simulink model "vRTHS_MDOF_SimRT"  (R2016a)
settings: Solver=ode4  StartTime=0.0  StopTime=tend  FixedStep=dt_rths  RelTol=1e-3
values from neighbouring files (symbols this model uses):
  a = 53354    [A3_Frequency_Response.m]    (also in F2_controller.m)
  a1_beta0 = 2.1283e+13    (= 21283000000000)    [F1_input_file.m]
  a2 = 4.23e6    (= 4230000)    [A3_Frequency_Response.m]    (also in F1_input_file.m = 4229700)
  a3 = [3.3-uncer*1.3,3.3+uncer*1.3]    [A3_Frequency_Response.m]    (also in F1_input_file.m = 3.3        + 1.3   * nom *randn(1,1))
  A_ns = [     zeros(n) eye(n) ... (first row only)    [F1_input_file.m]
  Ax = [0 1;-c -b]    [F2_controller.m]
  B_ns = [     zeros(n,1)      zeros(n) ... (first row only)    [F1_input_file.m]
  beta1 = 425        + 3.3   * nom *randn(1,1)    [F1_input_file.m]
  beta2 = 9.9976e+04 + 3.3e3 * nom *randn(1,1)    [F1_input_file.m]
  Bx = [0;1]    [F2_controller.m]
  C_ns = [     eye(n)              zeros(n) ... (first row only)    [F1_input_file.m]
  CE = zeros(n)    [F1_input_file.m]
  compd = [dt_rths 1]    [F2_controller.m]
  compn = [2*dt_rths 1]    [F2_controller.m]
  Cx = [1,0]    [F2_controller.m]
  d = 0.00010595    [A3_Frequency_Response.m]    (also in F2_controller.m)
  D_ns = [     zeros(n,1)      zeros(n) ... (first row only)    [F1_input_file.m]
  dt_rths = 1/fs    (= 0.000244140625)    [A1_main_SMC.m]    (also in A2_main_PI.m; A4_Plots.m)
  Dx = 0    [F2_controller.m]
  E_sw = 1    [A4_Plots.m]
  eq_intensity = .4    (= 0.4)    [A1_main_SMC.m]    (also in A2_main_PI.m; A4_Plots.m)
  Gsnsr_DT = 1    [F1_input_file.m]
  Gsnsr_FT = 1    [F1_input_file.m]
  KE = zeros(n)    [F1_input_file.m]
  ME = zeros(n)    [F1_input_file.m]
  Para = [b c b*bc c*cc lambda eta sw]    [F2_controller.m]
  Rx = rms_noise_DT/dt_rths    [F2_controller.m]
  Seed_snr = rng(seed)    [F1_input_file.m]
  tend = 90    [F1_input_file.m]
  xinitial = zeros(2,1)    [F2_controller.m]
undefined symbols (not defined in the file or in its folder): Continuous, Time
libraries: simulink x3, ctrlSharedLib x1, sldrtlib x1
settings Model: Creator=IISL_0175  LastModifiedBy=user
settings DataIOCC: SaveFormat=StructureWithTime
settings DebuggingCC: InheritedTsInSrcMsg=none
settings HardwareCC: ProdWordSize=32  ProdHWDeviceType=Specified

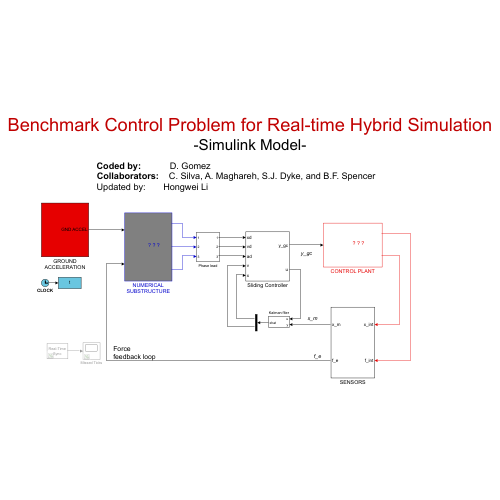
[thumbnail: Simulink's stored preview of the top-level diagram]
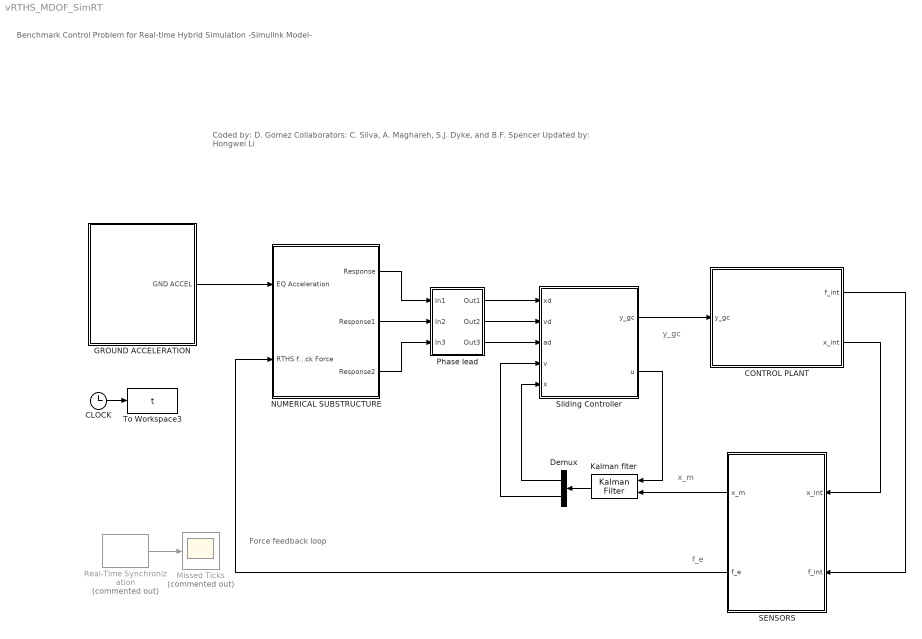
== system vRTHS_MDOF_SimRT ==
  note: Force
      | feedback loop
  note: Benchmark Control Problem for Real-time Hybrid Simulation
      | -Simulink Model-
  note: Coded by: D. Gomez
      | Collaborators: C. Silva, A. Maghareh, S.J. Dyke, and B.F. Spencer
      | Updated by: Hongwei Li
  note: y_gc
  note: f_e
  note: x_m
  CLOCK : Clock
  CONTROL PLANT : Subsystem
      mask Display: image(imread('PlantSW2.PNG'));
  Demux : Demux  Outputs=2
  GROUND ACCELERATION : Subsystem
  Kalman flter : ctrlSharedLib/Kalman Filter  TimeDomain=Continuous-Time  UseCurrentEstimator=on  ModelSource=Individual A, B, C, D matrices  ModelSourceVariable=ss(0.95,1,1,0,1)  A=Ax  B=Bx  C=Cx  D=Dx  NumberOfStates=2  NumberOfInputs=2  NumberOfOutputs=1  InitialEstimateSource=Dialog  X0=xinitial  P0=10  UseK=off  UseGH=off  NumberOfProcessNoiseInputs=1  G=1  TimeInvariantG=on  H=0  TimeInvariantH=on  Q=0  TimeInvariantQ=on  R=Rx  TimeInvariantR=on  N=0  TimeInvariantN=on  AddInputPort=on  AddEnablePort=off  OutputEstimatedY=off  OutputP=off  Ts=-1
  Missed Ticks : Scope  Commented=on
  NUMERICAL SUBSTRUCTURE : Subsystem
      mask Display: image(imread('Num_sub.png'));
  Phase lead : Subsystem
  Real-Time Synchronization : sldrtlib/Real-Time Synchronization  Commented=on  SampleTime=dt_rths  MaxMissedTicks=10000  ShowMissedTicks=on  YieldWhenWaiting=off
  SENSORS : Subsystem
  Sliding Controller : Subsystem
  To Workspace3 : ToWorkspace  VariableName=t  SampleTime=-1
  wires:
  CLOCK/1 -> To Workspace3/1
  CONTROL PLANT/2(x_int) -> SENSORS/1(x_int)
  Sliding Controller/1(y_gc) -> CONTROL PLANT/1(y_gc)
  Real-Time Synchronization/1 -> Missed Ticks/1
  GROUND ACCELERATION/1(GND ACCEL) -> NUMERICAL SUBSTRUCTURE/1(EQ Acceleration)
  CONTROL PLANT/1(f_int) -> SENSORS/2(f_int)
  SENSORS/2("f_e ") -> NUMERICAL SUBSTRUCTURE/2(RTHS feedback Force)
  NUMERICAL SUBSTRUCTURE/1(Response) -> Phase lead/1(In1)
  Phase lead/1(Out1) -> Sliding Controller/1(xd)
  Phase lead/2(Out2) -> Sliding Controller/2(vd)
  Phase lead/3(Out3) -> Sliding Controller/3(ad)
  NUMERICAL SUBSTRUCTURE/2(Response1) -> Phase lead/2(In2)
  NUMERICAL SUBSTRUCTURE/3(Response2) -> Phase lead/3(In3)
  Demux/1 -> Sliding Controller/5(x)
  Kalman flter/1 -> Demux/1
  SENSORS/1(x_m) -> Kalman flter/2
  Sliding Controller/2(u) -> Kalman flter/1
  Demux/2 -> Sliding Controller/4(v)

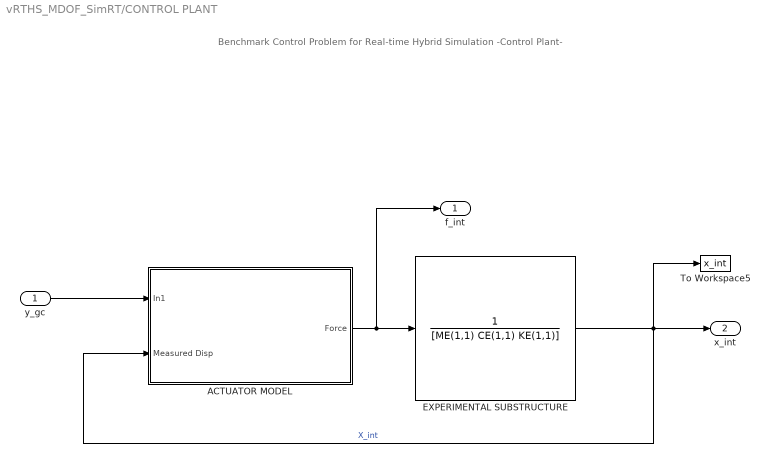
== system vRTHS_MDOF_SimRT/CONTROL PLANT ==
  note: Benchmark Control Problem for Real-time Hybrid Simulation
      | -Control Plant-
  y_gc : Inport
  ACTUATOR MODEL : Subsystem
      mask Display: image(imread('ActuatorSW2.PNG'));
  EXPERIMENTAL SUBSTRUCTURE : TransferFcn  Numerator=1  Denominator=[ME(1,1) CE(1,1) KE(1,1)]
      mask Display: image(imread('ESSW2.PNG'));
  To Workspace5 : ToWorkspace  VariableName=x_int  SampleTime=-1
  f_int : Outport
  x_int : Outport  Port=2
  wires:
  EXPERIMENTAL SUBSTRUCTURE/1 -> ACTUATOR MODEL/2(Measured Disp), To Workspace5/1, x_int/1  "X_int"
  ACTUATOR MODEL/1(Force) -> f_int/1, EXPERIMENTAL SUBSTRUCTURE/1
  y_gc/1 -> ACTUATOR MODEL/1(In1)

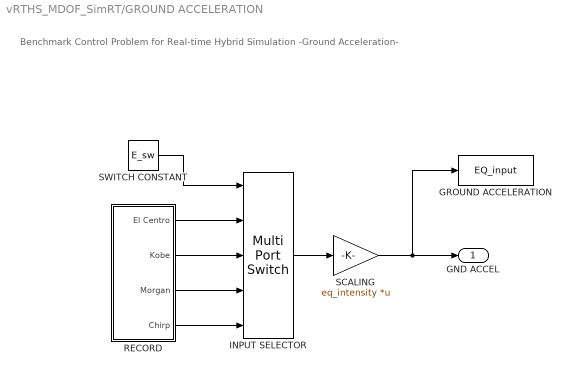
== system vRTHS_MDOF_SimRT/GROUND ACCELERATION ==
  note: Benchmark Control Problem for Real-time Hybrid Simulation
      | -Ground Acceleration-
  GROUND ACCELERATION : ToWorkspace  VariableName=EQ_input  SampleTime=-1
  INPUT SELECTOR : MultiPortSwitch  Inputs=4
  "RECORD " : Subsystem
  SCALING : Gain  Gain=eq_intensity  Multiplication=Matrix(K*u)
  SWITCH CONSTANT : Constant  Value=E_sw
  GND ACCEL : Outport
  wires:
  INPUT SELECTOR/1 -> SCALING/1
  SWITCH CONSTANT/1 -> INPUT SELECTOR/1
  "RECORD "/1(El Centro) -> INPUT SELECTOR/2
  "RECORD "/2(Kobe) -> INPUT SELECTOR/3
  "RECORD "/3(Morgan) -> INPUT SELECTOR/4
  SCALING/1 -> GROUND ACCELERATION/1, GND ACCEL/1
  "RECORD "/4(Chirp) -> INPUT SELECTOR/5

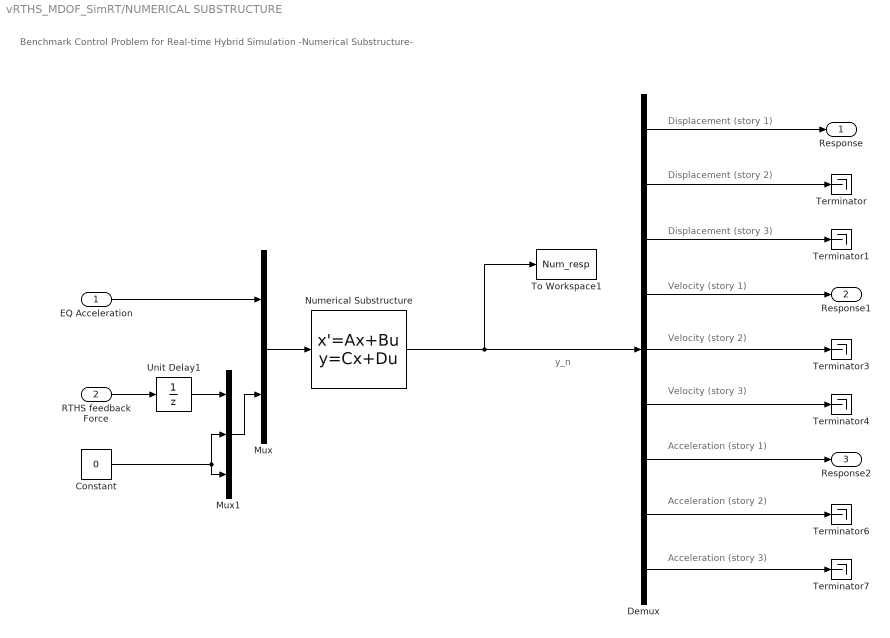
== system vRTHS_MDOF_SimRT/NUMERICAL SUBSTRUCTURE ==
  note: y_n
  note: Benchmark Control Problem for Real-time Hybrid Simulation
      | -Numerical Substructure-
  note: Velocity (story 3)
  note: Displacement (story 3)
  note: Displacement (story 1)
  note: Acceleration (story 1)
  note: Velocity (story 1)
  note: Velocity (story 2)
  note: Acceleration (story 3)
  note: Displacement (story 2)
  note: Acceleration (story 2)
  EQ Acceleration : Inport
  RTHS feedback Force : Inport  Port=2
  Constant : Constant  Value=0
  Demux : Demux  Outputs=9
  Mux : Mux  Inputs=2
  Mux1 : Mux  Inputs=3
  Numerical Substructure : StateSpace  A=A_ns  B=B_ns  C=C_ns  D=D_ns  X0=0
  Terminator{,1,3..4,6..7} (6 alike) : Terminator
  To Workspace1 : ToWorkspace  VariableName=Num_resp  SaveFormat=Timeseries  SampleTime=-1
  Unit Delay1 : UnitDelay  SampleTime=-1  HasFrameUpgradeWarning=on
  Response : Outport
  Response1 : Outport  Port=2
  Response2 : Outport  Port=3
  wires:
  Mux/1 -> Numerical Substructure/1
  EQ Acceleration/1 -> Mux/1
  RTHS feedback Force/1 -> Unit Delay1/1
  Numerical Substructure/1 -> To Workspace1/1, Demux/1
  Demux/2 -> Terminator/1
  Demux/7 -> Response2/1
  Demux/8 -> Terminator6/1
  Demux/9 -> Terminator7/1
  Demux/4 -> Response1/1
  Demux/6 -> Terminator4/1
  Demux/5 -> Terminator3/1
  Demux/1 -> Response/1
  Demux/3 -> Terminator1/1
  Constant/1 -> Mux1/2, Mux1/3
  Mux1/1 -> Mux/2
  Unit Delay1/1 -> Mux1/1

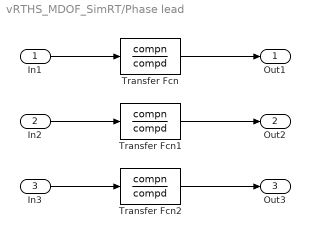
== system vRTHS_MDOF_SimRT/Phase lead ==
  In1 : Inport
  In2 : Inport  Port=2
  In3 : Inport  Port=3
  Transfer Fcn : TransferFcn  Numerator=compn  Denominator=compd
  Transfer Fcn1 : TransferFcn  Numerator=compn  Denominator=compd
  Transfer Fcn2 : TransferFcn  Numerator=compn  Denominator=compd
  Out1 : Outport
  Out2 : Outport  Port=2
  Out3 : Outport  Port=3
  wires:
  In1/1 -> Transfer Fcn/1
  Transfer Fcn/1 -> Out1/1
  In2/1 -> Transfer Fcn1/1
  Transfer Fcn1/1 -> Out2/1
  In3/1 -> Transfer Fcn2/1
  Transfer Fcn2/1 -> Out3/1

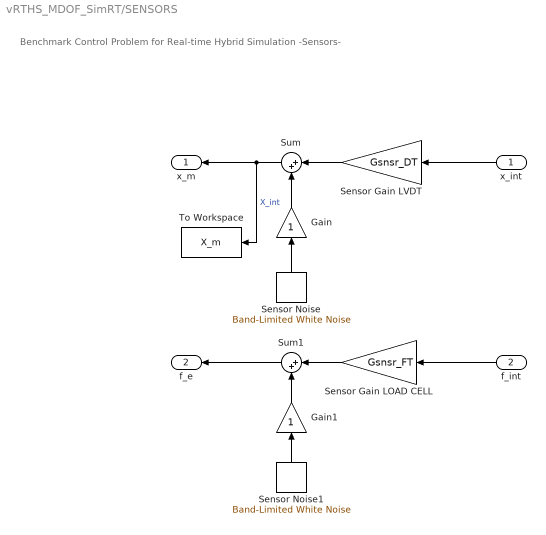
== system vRTHS_MDOF_SimRT/SENSORS ==
  note: Benchmark Control Problem for Real-time Hybrid Simulation
      | -Sensors-
  x_int : Inport
  f_int : Inport  Port=2
  Gain : Gain
  Gain1 : Gain
  Sensor Noise : simulink/Sources/Band-Limited White Noise  Cov=rms_noise_DT  Ts=dt_rths  seed=double(Seed_snr.Seed)
  Sensor Noise1 : simulink/Sources/Band-Limited White Noise  Cov=rms_noise_FT  Ts=dt_rths  seed=double(Seed_snr.Seed)
  Sensor Gain LVDT : Gain  Gain=Gsnsr_DT  SaturateOnIntegerOverflow=on  OutDataTypeStr=Inherit: Same as input  ParamDataTypeStr=Inherit: Same as input
  Sensor Gain LOAD CELL : Gain  Gain=Gsnsr_FT  SaturateOnIntegerOverflow=on  OutDataTypeStr=Inherit: Same as input  ParamDataTypeStr=Inherit: Same as input
  Sum : Sum  Inputs=|++  InputSameDT=on  SaturateOnIntegerOverflow=on  OutDataTypeStr=Inherit: Same as first input
  Sum1 : Sum  Inputs=|++  InputSameDT=on  SaturateOnIntegerOverflow=on  OutDataTypeStr=Inherit: Same as first input
  To Workspace : ToWorkspace  VariableName=X_m  SaveFormat=Timeseries  SampleTime=-1
  x_m : Outport
  "f_e " : Outport  Port=2
  wires:
  Sensor Gain LVDT/1 -> Sum/1
  Sensor Noise/1 -> Gain/1
  x_int/1 -> Sensor Gain LVDT/1
  Sensor Gain LOAD CELL/1 -> Sum1/1
  Sum1/1 -> "f_e "/1
  Sensor Noise1/1 -> Gain1/1
  f_int/1 -> Sensor Gain LOAD CELL/1
  Sum/1 -> x_m/1, To Workspace/1  "X_int"
  Gain/1 -> Sum/2
  Gain1/1 -> Sum1/2

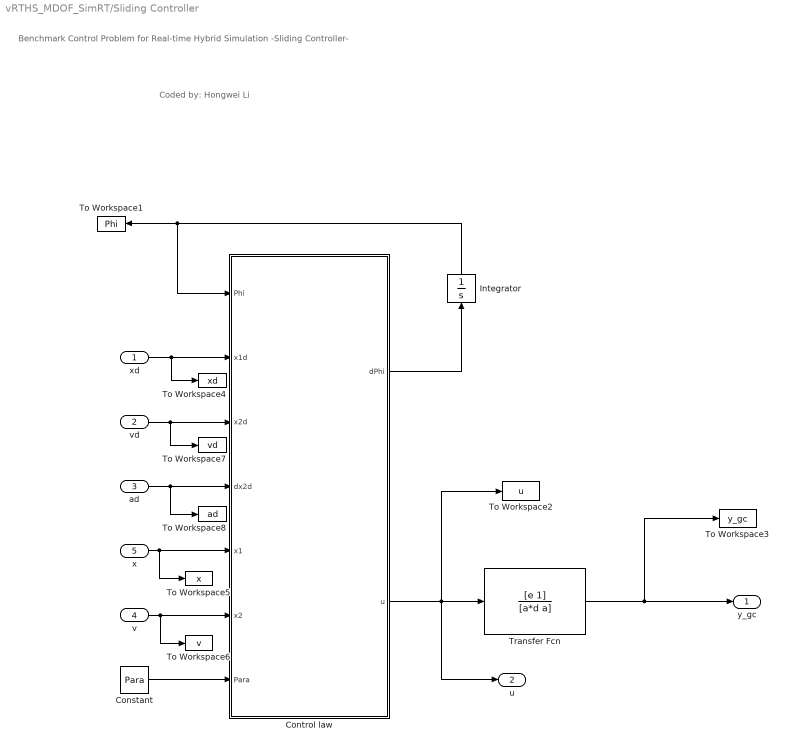
== system vRTHS_MDOF_SimRT/Sliding Controller ==
  note: Coded by: Hongwei Li
  note: Benchmark Control Problem for Real-time Hybrid Simulation
      | -Sliding Controller-
  xd : Inport
  vd : Inport  Port=2
  ad : Inport  Port=3
  v : Inport  Port=4
  x : Inport  Port=5
  Constant : Constant  Value=Para
  Control law : MATLAB Function  TreatAsAtomicUnit=on
  Integrator : Integrator
  To Workspace1 : ToWorkspace  VariableName=Phi  SampleTime=-1
  To Workspace2 : ToWorkspace  VariableName=u  SampleTime=-1
  To Workspace3 : ToWorkspace  VariableName=y_gc  SampleTime=-1
  To Workspace4 : ToWorkspace  VariableName=xd  SampleTime=-1
  To Workspace5 : ToWorkspace  VariableName=x  SampleTime=-1
  To Workspace6 : ToWorkspace  VariableName=v  SampleTime=-1
  To Workspace7 : ToWorkspace  VariableName=vd  SampleTime=-1
  To Workspace8 : ToWorkspace  VariableName=ad  SampleTime=-1
  Transfer Fcn : TransferFcn  Numerator=[e 1]  Denominator=[a*d a]
  y_gc : Outport
  u : Outport  Port=2
  wires:
  ad/1 -> To Workspace8/1, Control law/4(dx2d)
  vd/1 -> Control law/3(x2d), To Workspace7/1
  x/1 -> To Workspace5/1, Control law/5(x1)
  Constant/1 -> Control law/7(Para)
  Integrator/1 -> To Workspace1/1, Control law/1(Phi)
  v/1 -> To Workspace6/1, Control law/6(x2)
  xd/1 -> Control law/2(x1d), To Workspace4/1
  Control law/1(dPhi) -> Integrator/1
  Transfer Fcn/1 -> y_gc/1, To Workspace3/1
  Control law/2(u) -> u/1, To Workspace2/1, Transfer Fcn/1

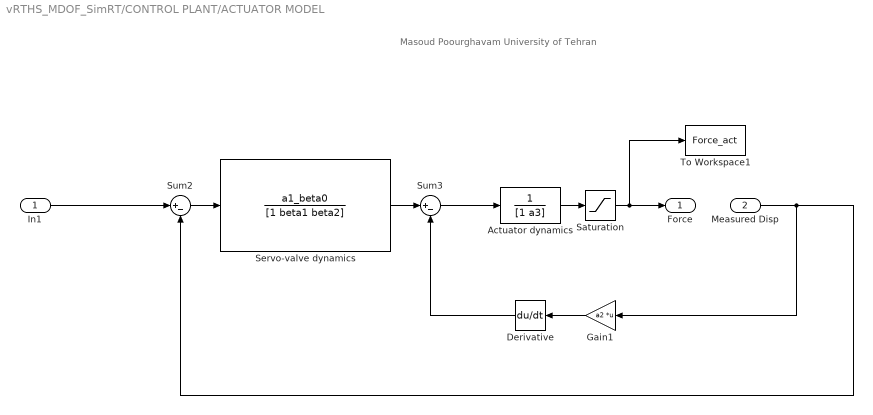
== system vRTHS_MDOF_SimRT/CONTROL PLANT/ACTUATOR MODEL ==
  note: Masoud Poourghavam
      | University of Tehran
  In1 : Inport
  Measured Disp : Inport  Port=2
  Actuator dynamics : TransferFcn  Numerator=1  Denominator=[1 a3]
  Derivative : Derivative
  Gain1 : Gain  Gain=a2  Multiplication=Matrix(K*u)
  Saturation : Saturate  UpperLimit=8900  LowerLimit=-8900
  Servo-valve dynamics : TransferFcn  Numerator=a1_beta0  Denominator=[1 beta1 beta2]
  Sum2 : Sum  Inputs=|+-
  Sum3 : Sum  Inputs=|+-
  To Workspace1 : ToWorkspace  VariableName=Force_act  SampleTime=-1
  Force : Outport
  wires:
  In1/1 -> Sum2/1
  Actuator dynamics/1 -> Saturation/1
  Servo-valve dynamics/1 -> Sum3/1
  Sum2/1 -> Servo-valve dynamics/1
  Gain1/1 -> Derivative/1
  Derivative/1 -> Sum3/2
  Sum3/1 -> Actuator dynamics/1
  Measured Disp/1 -> Sum2/2, Gain1/1
  Saturation/1 -> To Workspace1/1, Force/1

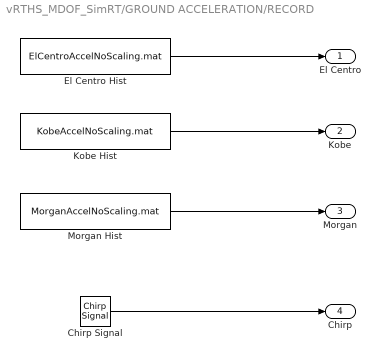
== system vRTHS_MDOF_SimRT/GROUND ACCELERATION/RECORD  ==
  Chirp Signal : simulink/Sources/Chirp Signal  f1=f_ini  T=tend  f2=f_end
  El Centro Hist : FromFile  FileName=ElCentroAccelNoScaling.mat
  Kobe Hist : FromFile  FileName=KobeAccelNoScaling.mat
  Morgan Hist : FromFile  FileName=MorganAccelNoScaling.mat
  El Centro : Outport
  Kobe : Outport  Port=2
  Morgan : Outport  Port=3
  Chirp : Outport  Port=4
  wires:
  Morgan Hist/1 -> Morgan/1
  Kobe Hist/1 -> Kobe/1
  El Centro Hist/1 -> El Centro/1
  Chirp Signal/1 -> Chirp/1

== matlab function vRTHS_MDOF_SimRT/Sliding Controller/Control law ==
  data: Phi input; dPhi output; x1d input; x2d input; dx2d input; x1 input; x2 input; Para input; u output
function [dPhi,u]  = Controller(Phi,x1d,x2d,dx2d,x1,x2,Para)
bbar=Para(1); cbar=Para(2);
bM=Para(3); cM=Para(4);
lambda=Para(5); eta=Para(6);
sw=Para(7);

fbar=-bbar*x2-cbar*x1;
ubar=-fbar+dx2d-lambda*(x2-x2d);
F=bM*abs(x2)+cM*abs(x1);
k=F+eta;
Fd=bM*abs(x2d)+cM*abs(x1d);
dPhi=Fd+eta-lambda*Phi;
kbar=k-dPhi;
E=x2-x2d+lambda*(x1-x1d);
if sw==1
    if abs(E)>=Phi
        sat=sign(E);
    else
        sat=E/Phi;
    end
else
    sat=sign(E);
    dPhi=0;
    kbar=k;
end
u=ubar-kbar*sat;
